simulink model "Inverter1_1"  (R2013a)
settings: Solver=ode45  StartTime=0.0  StopTime=5/50  RelTol=1e-3
libraries: powerlib x17, simulink x5
settings Model: Creator=HP6k  LastModifiedBy=HP6k

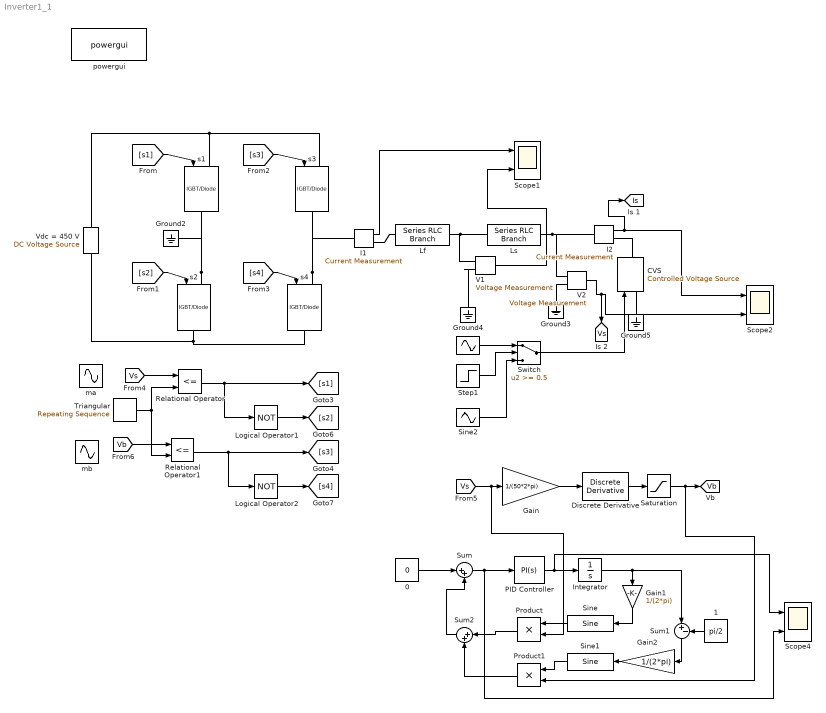
== system Inverter1_1 ==
  " " : Sin  Amplitude=311  Frequency=2*pi*50  SampleTime=0
  0 : Constant  Value=0
  "1 " : Constant  Value=pi/2
  CVS : powerlib/Electrical Sources/Controlled Voltage Source  Initialize=on  Source_Type=AC  Amplitude=311  Phase=0  Frequency=50  Measurements=None
  Discrete Derivative : simulink/Discrete/Discrete Derivative  gainval=1.0  ICPrevScaledInput=0.0  InputProcessing=Inherited  OutMin=[]  OutMax=[]  OutDataType=fixdt(1, 16)  OutScaling=2^-10  DoSatur=off
  Gain : Gain  Gain=1/(50*2*pi)
  Gain1 : Gain  Gain=1/(2*pi)
  Gain2 : Gain  Gain=1/(2*pi)
  Ground{2..5} (4 alike) : powerlib/Elements/Ground  LConnTagsString=a
  I1 : powerlib/Measurements/Current Measurement  Tag=PoWeRsYsTeMmEaSuReMeNt  PhasorSimulation=off  OutputType=Magnitude  PSBequivalent=0
  I2 : powerlib/Measurements/Current Measurement  Tag=PoWeRsYsTeMmEaSuReMeNt  PhasorSimulation=off  OutputType=Magnitude  PSBequivalent=0
  Integrator : Integrator
  Lf : powerlib/Elements/Series RLC Branch  LConnTagsString=__new0  RConnTagsString=__new0  BranchType=RL  Resistance=1  Inductance=2e-3  SetiL0=off  InitialCurrent=0  Capacitance=1e-6  Setx0=off  InitialVoltage=0  Measurements=None
  Logical Operator1 : Logic  Operator=NOT  AllPortsSameDT=off  OutDataTypeStr=boolean
  Logical Operator2 : Logic  Operator=NOT  AllPortsSameDT=off  OutDataTypeStr=boolean
  Ls : powerlib/Elements/Series RLC Branch  LConnTagsString=__new0  RConnTagsString=__new0  BranchType=RL  Resistance=1  Inductance=1.5e-3  SetiL0=off  InitialCurrent=0  Capacitance=1e-6  Setx0=off  InitialVoltage=0  Measurements=None
  PID Controller : simulink/Continuous/PID Controller  Controller=PI  TimeDomain=Continuous-time  SampleTime=1  IntegratorMethod=Forward Euler  FilterMethod=Forward Euler  Form=Parallel  P=10  I=10  D=0  N=100  InitialConditionSource=internal  InitialConditionForIntegrator=0  InitialConditionForFilter=0  ExternalReset=none  LimitOutput=off  UpperSaturationLimit=inf  LowerSaturationLimit=-inf  LinearizeAsGain=on  AntiWindupMode=none  Kb=1  TrackingMode=off  Kt=1  PParamMin=[]  PParamMax=[]  IParamMin=[]  IParamMax=[]  DParamMin=[]  DParamMax=[]  NParamMin=[]  NParamMax=[]  KbParamMin=[]  KbParamMax=[]  KtParamMin=[]  KtParamMax=[]  POutMin=[]  POutMax=[]  IOutMin=[]  IOutMax=[]  DOutMin=[]  DOutMax=[]  NOutMin=[]  NOutMax=[]  KbOutMin=[]  KbOutMax=[]  KtOutMin=[]  KtOutMax=[]  IntegratorOutMin=[]  IntegratorOutMax=[]  FilterOutMin=[]  FilterOutMax=[]  SumOutMin=[]  SumOutMax=[]  SumI1OutMin=[]  SumI1OutMax=[]  SumI2OutMin=[]  SumI2OutMax=[]  SumI3OutMin=[]  SumI3OutMax=[]  SumDOutMin=[]  SumDOutMax=[]  SaturationOutMin=[]  SaturationOutMax=[]  IntegratorContinuousStateAttributes=''  IntegratorStateMustResolveToSignalObject=off  IntegratorRTWStateStorageClass=Auto  FilterContinuousStateAttributes=''  FilterStateMustResolveToSignalObject=off  FilterRTWStateStorageClass=Auto
  Product : Product
  Product1 : Product
  Relational Operator : RelationalOperator  Operator=<=  OutDataTypeStr=boolean
  Relational Operator1 : RelationalOperator  Operator=<=  OutDataTypeStr=boolean
  Saturation : Saturate  UpperLimit=312  LowerLimit=-312
  Scope1 : Scope  NumInputPorts=2
      settings: TimeRange=0.1  YMin=-100~-300  YMax=100~300  SaveName=sps1phPWM1_str1  MaxDataPoints=500000
  Scope2 : Scope  NumInputPorts=2
      settings: TimeRange=0.1  YMin=-100~-300  YMax=100~300  SaveName=sps1phPWM1_str  MaxDataPoints=500000
  Scope4 : Scope  NumInputPorts=2
      settings: TimeRange=0.1  YMin=-100~-300  YMax=100~300  SaveName=sps1phPWM1_str3  MaxDataPoints=500000
  Sine : simulink/Lookup Tables/Sine  Formula=sin(2*pi*u)  NumDataPoints=(2^5)+1  OutputWordLength=16
  Sine1 : simulink/Lookup Tables/Sine  Formula=sin(2*pi*u)  NumDataPoints=(2^5)+1  OutputWordLength=16
  "Sine2 " : Sin  Amplitude=311  Frequency=2*pi*100  SampleTime=0
  Step1 : Step  Time=2/50  Before=1  After=0  SampleTime=0
  Sum : Sum  Inputs=|++
  Sum1 : Sum  Inputs=|+-
  Sum2 : Sum  Inputs=|++
  Switch : Switch  Threshold=0.5  SaturateOnIntegerOverflow=on  InputSameDT=on
  Triangular : simulink/Sources/Repeating Sequence  rep_seq_t=[0 0.5 1]*1/10E3  rep_seq_y=[-1 1 -1]
  V1 : powerlib/Measurements/Voltage Measurement  Tag=PoWeRsYsTeMmEaSuReMeNt  PhasorSimulation=off  OutputType=Magnitude  PSBequivalent=0
  V2 : powerlib/Measurements/Voltage Measurement  Tag=PoWeRsYsTeMmEaSuReMeNt  PhasorSimulation=off  OutputType=Magnitude  PSBequivalent=0
  Vdc = 450 V : powerlib/Electrical Sources/DC Voltage Source  Description=source block  Amplitude=450  Measurements=None
      settings: AttributesFormatString=\n
  ma : Sin  Amplitude=0.8  Frequency=2*pi*50  SampleTime=0
  mb : Sin  Amplitude=0.8  Frequency=2*pi*50  Phase=-2*pi/3  SampleTime=0
  powergui : powerlib/powergui  Priority=1  SimulationMode=Discrete  SolverType=Backward Euler  SampleTime=1e-6  frequency=60  SPID=off  DisableSnubberDevices=off  DisableRonSwitches=off  DisableVfSwitches=off  SwTol=0  Interpol=off  DisplayEquations=off  frequencyindice=0  Pbase=100e6  ErrMax=1e-4  Iterations=50  UnitsV=kV  UnitsW=MW  FunctionMessages=off  echomessages=off  HookPort=off  EnableUseOfTLC=off  x0status=blocks  RestoreLinks=warning  ResistiveCurrentMeasurement=off  Frange=[0:2:500]  Ylog=off  Xlog=on  ShowGrid=off  save=off  variable=ZData  ZoomFFT=off  StartTime=0.0  cycles=1  DisplayStyle=1  fundamental=60  FreqAxis=off  MaxFrequency=1000  frequencyindicesteady=1  RmsSteady=1  display=off  Ts=0  methode=off
  s{1..4} (4 alike) : powerlib/Power Electronics/IGBT//Diode  Ron=1e-4  Rs=1e5  Cs=inf  Measurements=off
  tag scope: Is=global, Vb=global, Vs=global
  wires:
  Relational Operator/1 -> Logical Operator1/1, [s1]
  Logical Operator1/1 -> [s2]
  Triangular/1 -> Relational Operator1/2, Relational Operator/2
  Logical Operator2/1 -> [s4]
  Relational Operator1/1 -> Logical Operator2/1, [s3]
  [s2] -> s2/1
  [s3] -> s3/1
  [s1] -> s1/1
  [s4] -> s4/1
  I1/1 -> Scope1/1
  V2/1 -> [Vs], Scope2/2
  I2/1 -> [Is], Scope2/1
  V1/1 -> Scope1/2
  Step1/1 -> Switch/2
  " "/1 -> Switch/1
  "Sine2 "/1 -> Switch/3
  Switch/1 -> CVS/1
  [Vs] -> Product/2, Gain/1
  Discrete Derivative/1 -> Saturation/1
  Gain/1 -> Discrete Derivative/1
  Saturation/1 -> Product1/2, [Vb]
  [Vs] -> Relational Operator/1
  [Vb] -> Relational Operator1/1
  PID Controller/1 -> Integrator/1, Scope4/1
  Sum/1 -> Scope4/2, PID Controller/1
  Integrator/1 -> Gain1/1, Sum1/1
  "1 "/1 -> Sum1/2
  Gain1/1 -> Sine/1
  Gain2/1 -> Sine1/1
  Sum1/1 -> Gain2/1
  Sine/1 -> Product/1
  Sine1/1 -> Product1/1
  Product/1 -> Sum2/1
  Product1/1 -> Sum2/2
  Sum2/1 -> Sum/2
  0/1 -> Sum/1
  connections:
  s4/LConn1 -- s3/RConn1 -- I1/LConn1
  s2/RConn1 -- s4/RConn1 -- Vdc = 450 V/LConn1
  s2/LConn1 -- s1/RConn1 -- Ground2/LConn1
  Vdc = 450 V/RConn1 -- s1/LConn1 -- s3/LConn1
  V1/LConn1 -- Ls/LConn1 -- Lf/RConn1
  Ls/RConn1 -- I2/LConn1 -- V2/LConn1
  I1/RConn1 -- Lf/LConn1
  V1/LConn2 -- Ground4/LConn1
  CVS/LConn1 -- Ground5/LConn1
  V2/LConn2 -- Ground3/LConn1
  CVS/RConn1 -- I2/RConn1
